simulink library "TBMPC_Blocks"  (R2020a)
settings: Solver=VariableStepAuto  StartTime=0.0  StopTime=10.0  RelTol=1e-3
settings Model: Creator=hough  LastModifiedBy=jeffh

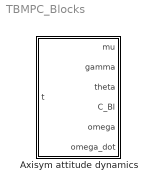
== system TBMPC_Blocks ==
  Axisym attitude dynamics : Subsystem  mask{J_transverse=0, J_z=0, omega_t=0, omega_z=0, mu_0=0, gamma_0=0, theta_0=0}
      mask prompts: J_transverse "Inertia (transverse)"; J_z "Inertia (sym axis)"; omega_t "Angular vel (trans axis)"; omega_z "Angular vel (sym axis)"; mu_0 "Initial mu angle"; gamma_0 "Initial gamma angle"; theta_0 "Initial theta angle"
      mask help: This block performs the attitude dynamics for an axi symmetric target spacecraft assuming 0 distrubances.

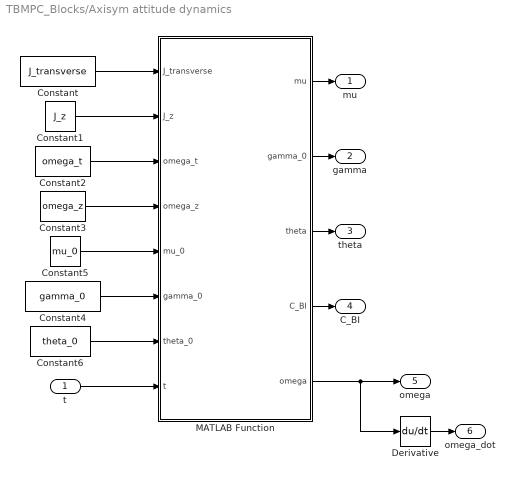
== system TBMPC_Blocks/Axisym attitude dynamics ==
  t : Inport
  Constant : Constant  Value=J_transverse
  Constant1 : Constant  Value=J_z
  Constant2 : Constant  Value=omega_t
  Constant3 : Constant  Value=omega_z
  Constant4 : Constant  Value=gamma_0
  Constant5 : Constant  Value=mu_0
  Constant6 : Constant  Value=theta_0
  Derivative : Derivative
  MATLAB Function : MATLAB Function  TreatAsAtomicUnit=on
  mu : Outport
  gamma : Outport  Port=2
  theta : Outport  Port=3
  C_BI : Outport  Port=4
  omega : Outport  Port=5
  omega_dot : Outport  Port=6
  wires:
  t/1 -> MATLAB Function/8(t)
  MATLAB Function/1(mu) -> mu/1
  Constant/1 -> MATLAB Function/1(J_transverse)
  Constant1/1 -> MATLAB Function/2(J_z)
  Constant2/1 -> MATLAB Function/3(omega_t)
  Constant3/1 -> MATLAB Function/4(omega_z)
  Constant4/1 -> MATLAB Function/6("gamma_0 ")
  Constant5/1 -> MATLAB Function/5(mu_0)
  Constant6/1 -> MATLAB Function/7(theta_0)
  MATLAB Function/2(gamma_0) -> gamma/1
  MATLAB Function/3(theta) -> theta/1
  MATLAB Function/4(C_BI) -> C_BI/1
  MATLAB Function/5(omega) -> Derivative/1, omega/1
  Derivative/1 -> omega_dot/1

== matlab function TBMPC_Blocks/Axisym attitude dynamics/MATLAB Function ==
  data: J_transverse input; mu output; J_z input; omega_t input; omega_z input; mu_0 input; gamma_0 input; theta_0 input; t input; gamma_0 output; theta output; C_BI output; omega output
function [mu, gamma_0, theta, C_BI, omega] = fcn(J_transverse, J_z, omega_t, omega_z, mu_0, gamma_0, theta_0, t)
        
    % First, solve for captital omega:
    mu_dot = (J_transverse - J_z)/J_transverse * omega_z;
    
    % Get the total momentum:
    h = sqrt((J_z*omega_z)^2 + (J_transverse*omega_t)^2);
    
    % Solve for the rate of precession:
    theta_dot = h/J_transverse;
    
    % solve for the upcoming angles:
    mu = mu_0 + mu_dot*t;
    theta = theta_0 + theta_dot * t;
    
    % Solve for the new rotation matrix:
    C_BI =  C3(mu)*C1(gamma_0)*C3(theta);

    % Solve for the new angular velocity:
    omega = [theta_dot*sin(gamma_0)*sin(mu);
             theta_dot*sin(gamma_0)*cos(mu);
             mu_dot + theta_dot*cos(gamma_0)];
    
end
